simulink model "ThreeWheeledVehicle"  (R2017b)
settings: Solver=VariableStepAuto  StartTime=0.0  StopTime=25  RelTol=1e-3
undefined symbols (not defined in the file): b_contact_RW, C_F_alpha, C_F_kappa, CM_phi, Cylinder, Dtheta0, epsilon, g, k_contact_RW, lengthRW, massRW, Parts_Lib, radiusRW, sigbuilder_block, sigma, X, xPla, Y, yPla, Z, zPla
libraries: nesl_utility x42, sm_lib x39, vrlib x21, simulink x3
(part 3 of 3)

== system ThreeWheeledVehicle/Tire model1/Lateral Force A ==
  v_cx : Inport
  alpha : Inport  Port=2
  eLat : Inport  Port=3
  Constant : Constant  Value=sigma
  Constant1 : Constant  Value=sigma
  Gain : Gain  Gain=-C_F_alpha
  Integrator : Integrator
  Product{,1..4} (5 alike) : Product
  Scope : Scope
  Scope1 : Scope
  Sum : Sum  Inputs=|+-
  v_cx1 : InportShadow
  Fz : Outport
  wires:
  alpha/1 -> Scope1/1, Product/1  "input"
  v_cx/1 -> Product1/1
  Product/1 -> Sum/1
  Product1/1 -> Product/2
  Constant/1 -> Product1/2
  Sum/1 -> Integrator/1
  Integrator/1 -> Gain/1, Product2/1  "output"
  v_cx1/1 -> Product3/1
  Constant1/1 -> Product3/2
  Product3/1 -> Product2/2
  Product2/1 -> Sum/2
  Gain/1 -> Product4/1
  eLat/1 -> Product4/2
  Product4/1 -> Scope/1, Fz/1

== system ThreeWheeledVehicle/Tire model1/Lateral slip with relaxation ==
  v_s : Inport
  eLat : Inport  Port=2
  v_cx : Inport  Port=3
  eLong : Inport  Port=4
  Dot Product : DotProduct  InputSameDT=on  OutDataTypeStr=Inherit: Inherit via internal rule
  Gain : Gain  Gain=1/sigma
  Gain1 : Gain  Gain=-C_F_alpha
  Integrator : Integrator
  Product : Product
  Product1 : Product
  Scope : Scope
  Scope1 : Scope
  Scope2 : Scope
  Sum : Sum  Inputs=|+-
  F_Lat : Outport
  wires:
  v_s/1 -> Dot Product/1
  eLat/1 -> Product1/2, Dot Product/2
  Dot Product/1 -> Scope1/1, Sum/1  "s2"
  Product/1 -> Sum/2
  Sum/1 -> Gain/1
  Gain/1 -> Integrator/1
  Integrator/1 -> Scope2/1, Gain1/1, Product/2  "alpha_F"
  Gain1/1 -> Product1/1
  Product1/1 -> Scope/1, F_Lat/1
  v_cx/1 -> Product/1

== system ThreeWheeledVehicle/Tire model1/Longitudinal Force A ==
  v_cx : Inport
  kappa : Inport  Port=2
  eLong : Inport  Port=3
  Constant : Constant  Value=sigma
  Constant1 : Constant  Value=sigma
  Gain : Gain  Gain=-C_F_kappa
  Integrator : Integrator
  Product{,1..4} (5 alike) : Product
  Scope : Scope
  Scope1 : Scope
  Sum : Sum  Inputs=|+-
  v_cx1 : InportShadow
  Fx : Outport
  wires:
  kappa/1 -> Scope1/1, Product/1  "input"
  v_cx/1 -> Product1/1
  Product/1 -> Sum/1
  Product1/1 -> Product/2
  Constant/1 -> Product1/2
  Sum/1 -> Integrator/1
  Integrator/1 -> Gain/1, Product2/1  "output"
  v_cx1/1 -> Product3/1
  Constant1/1 -> Product3/2
  Product3/1 -> Product2/2
  Product2/1 -> Sum/2
  Gain/1 -> Product4/1
  eLong/1 -> Product4/2
  Product4/1 -> Scope/1, Fx/1

== system ThreeWheeledVehicle/Tire model1/Longitudinal slip with relaxation ==
  v_s : Inport
  eLong : Inport  Port=2
  v_cx : Inport  Port=3
  Dot Product : DotProduct  InputSameDT=on  OutDataTypeStr=Inherit: Inherit via internal rule
  Gain : Gain  Gain=1/sigma
  Gain1 : Gain  Gain=-C_F_kappa
  Integrator : Integrator
  Product : Product
  Product1 : Product
  Scope : Scope
  Scope1 : Scope
  Sum : Sum  Inputs=|+-
  F_Long : Outport
  wires:
  v_s/1 -> Dot Product/1
  eLong/1 -> Product1/2, Dot Product/2
  Dot Product/1 -> Scope1/1, Sum/1  "s1"
  Product/1 -> Sum/2
  Sum/1 -> Gain/1
  Gain/1 -> Integrator/1
  Integrator/1 -> Gain1/1, Product/2  "kappa_F"
  Gain1/1 -> Product1/1
  Product1/1 -> Scope/1, F_Long/1
  v_cx/1 -> Product/1

== system ThreeWheeledVehicle/Tire model1/Sensing ==
  PS-Simulink Converter{,1..9} (10 alike) : nesl_utility/PS-Simulink Converter  PhysicalDomain=network_engine_domain  SubClassName=ps_output  LeftPortType=input  RightPortType=output  PseudoPeriodic=off  Frequencies=[]  Unit=1  AffineConversion=off
  Scope : Scope
  Transform Sensor : sm_lib/Frames and Transforms/Transform Sensor  MeasurementFrame=Base  SenseAngle=off  SenseAxis=off  SenseAngle1=off  SenseAngle2=off  SenseAngle3=off  SenseQ=off  SenseR=on  SenseOmegaX=on  SenseOmegaY=on  SenseOmegaZ=on  SenseOmega1=off  SenseOmega2=off  SenseOmega3=off  SenseQDot=off  SenseRDot=off  SenseAlphaX=off  SenseAlphaY=off  SenseAlphaZ=off  SenseAlpha1=off  SenseAlpha2=off  SenseAlpha3=off  SenseQDDot=off  SenseRDDot=off  SenseX=on  SenseY=on  SenseZ=on  SenseRad=off  SenseAzim=off  SenseDist=off  SenseInc=off  SenseXDot=on  SenseYDot=on  SenseZDot=on  SenseRadDot=off  SenseAzimDot=off  SenseDistDot=off  SenseIncDot=off  SenseXDDot=off  SenseYDDot=off  SenseZDDot=off  SenseRadDDot=off  SenseAzimDDot=off  SenseDistDDot=off  SenseIncDDot=off
  Wheel : PMIOPort  Port=1  Side=Left
  Plane : PMIOPort  Port=2  Side=Left
  R : Outport
  x : Outport  Port=2
  y : Outport  Port=3
  z : Outport  Port=4
  vx : Outport  Port=5
  vy : Outport  Port=6
  vz : Outport  Port=7
  wx : Outport  Port=8
  wy : Outport  Port=9
  wz : Outport  Port=10
  wires:
  PS-Simulink Converter2/1 -> wy/1
  PS-Simulink Converter8/1 -> vy/1
  PS-Simulink Converter9/1 -> vz/1
  PS-Simulink Converter1/1 -> wx/1
  PS-Simulink Converter4/1 -> x/1
  PS-Simulink Converter7/1 -> vx/1
  PS-Simulink Converter3/1 -> wz/1
  PS-Simulink Converter5/1 -> y/1
  PS-Simulink Converter6/1 -> Scope/1, z/1
  PS-Simulink Converter/1 -> R/1
  connections:
  PS-Simulink Converter1/LConn1 -- Transform Sensor/RConn3
  PS-Simulink Converter4/LConn1 -- Transform Sensor/RConn6
  PS-Simulink Converter3/LConn1 -- Transform Sensor/RConn5
  PS-Simulink Converter9/LConn1 -- Transform Sensor/RConn11
  PS-Simulink Converter2/LConn1 -- Transform Sensor/RConn4
  PS-Simulink Converter6/LConn1 -- Transform Sensor/RConn8
  PS-Simulink Converter/LConn1 -- Transform Sensor/RConn2
  Transform Sensor/LConn1 -- Plane/RConn1
  Transform Sensor/RConn1 -- Wheel/RConn1
  PS-Simulink Converter5/LConn1 -- Transform Sensor/RConn7
  PS-Simulink Converter7/LConn1 -- Transform Sensor/RConn9
  PS-Simulink Converter8/LConn1 -- Transform Sensor/RConn10

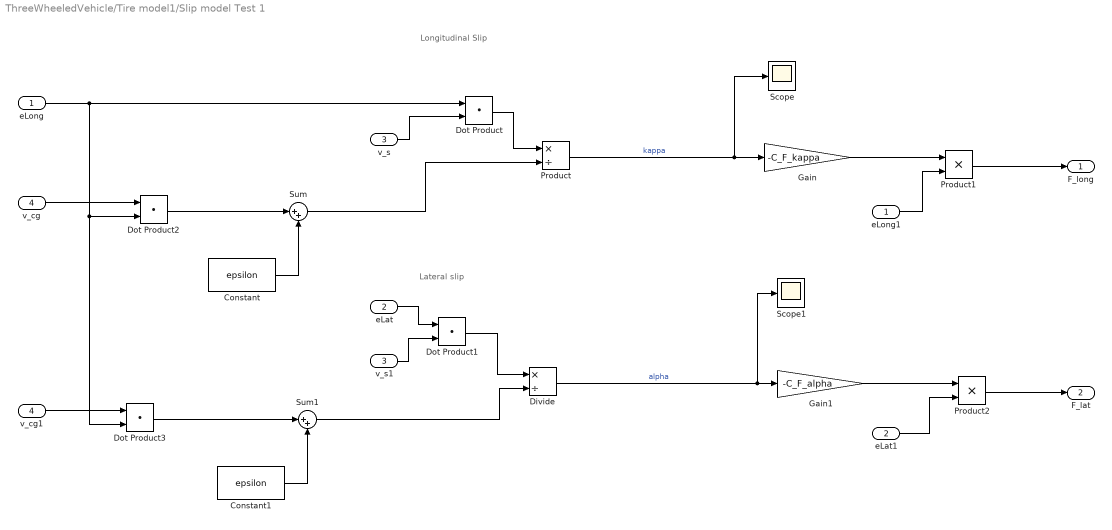
== system ThreeWheeledVehicle/Tire model1/Slip model Test 1 ==
  note: Lateral slip
  note: Longitudinal Slip
  eLong : Inport
  eLat : Inport  Port=2
  v_s : Inport  Port=3
  v_cg : Inport  Port=4
  Constant : Constant  Value=epsilon
  Constant1 : Constant  Value=epsilon
  Divide : Product  Inputs=*/
  Dot Product{,1..3} (4 alike) : DotProduct  InputSameDT=on  OutDataTypeStr=Inherit: Inherit via internal rule
  Gain : Gain  Gain=-C_F_kappa
  Gain1 : Gain  Gain=-C_F_alpha
  Product : Product  Inputs=*/
  Product1 : Product
  Product2 : Product
  Scope : Scope
  Scope1 : Scope
  Sum : Sum  Inputs=|++
  Sum1 : Sum  Inputs=|++
  eLat1 : InportShadow  Port=2
  eLong1 : InportShadow
  v_cg1 : InportShadow  Port=4
  v_s1 : InportShadow  Port=3
  F_long : Outport
  F_lat : Outport  Port=2
  wires:
  eLong/1 -> Dot Product3/2, Dot Product2/2, Dot Product/1
  v_s/1 -> Dot Product/2
  Dot Product/1 -> Product/1
  Product/1 -> Scope/1, Gain/1  "kappa"
  eLat/1 -> Dot Product1/1
  v_s1/1 -> Dot Product1/2
  Dot Product1/1 -> Divide/1
  Divide/1 -> Scope1/1, Gain1/1  "alpha"
  Gain/1 -> Product1/1
  eLong1/1 -> Product1/2
  Gain1/1 -> Product2/1
  eLat1/1 -> Product2/2
  Product1/1 -> F_long/1
  Product2/1 -> F_lat/1
  Constant/1 -> Sum/2
  Sum/1 -> Product/2
  Constant1/1 -> Sum1/2
  Sum1/1 -> Divide/2
  v_cg/1 -> Dot Product2/1
  Dot Product2/1 -> Sum/1
  v_cg1/1 -> Dot Product3/1
  Dot Product3/1 -> Sum1/1

== system ThreeWheeledVehicle/Tire model1/Slip model Test 2 ==
  note: Lateral slip
  note: Longitudinal Slip
  eLong : Inport
  eLat : Inport  Port=2
  v_s : Inport  Port=3
  v_cx : Inport  Port=4
  Divide : Product  Inputs=*/
  Dot Product : DotProduct  InputSameDT=on  OutDataTypeStr=Inherit: Inherit via internal rule
  Dot Product1 : DotProduct  InputSameDT=on  OutDataTypeStr=Inherit: Inherit via internal rule
  Gain : Gain  Gain=-C_F_kappa
  Gain1 : Gain  Gain=-C_F_alpha
  Product : Product  Inputs=*/
  Product1 : Product
  Product2 : Product
  Scope : Scope
  Scope1 : Scope
  eLat1 : InportShadow  Port=2
  eLong1 : InportShadow
  v_cx1 : InportShadow  Port=4
  v_s1 : InportShadow  Port=3
  F_long : Outport
  F_lat : Outport  Port=2
  kappa : Outport  Port=3
  alpha : Outport  Port=4
  wires:
  eLong/1 -> Dot Product/1
  Dot Product/1 -> Product/1
  eLat/1 -> Dot Product1/1
  Dot Product1/1 -> Divide/1
  Divide/1 -> alpha/1, Scope1/1, Gain1/1  "alpha"
  Gain/1 -> Product1/1
  eLong1/1 -> Product1/2
  Gain1/1 -> Product2/1
  eLat1/1 -> Product2/2
  Product1/1 -> F_long/1
  Product2/1 -> F_lat/1
  v_s/1 -> Dot Product/2
  v_s1/1 -> Dot Product1/2
  Product/1 -> Scope/1, kappa/1, Gain/1  "kappa"
  v_cx/1 -> Divide/2, Product/2

== system ThreeWheeledVehicle/Tire model1/Slip velocity ==
  omega : Inport
  v_cg : Inport  Port=2
  r : Inport  Port=3
  Add : Sum
  Cross Product : vrlib/Utilities/Cross Product
      settings: SourceProductBaseCode=VR
  Scope : Scope
  Scope1 : Scope
  Scope4 : Scope
  v_s : Outport
  wires:
  omega/1 -> Cross Product/1
  Cross Product/1 -> Scope/1, Add/2  "v_r"
  r/1 -> Cross Product/2
  Add/1 -> Scope4/1, v_s/1
  v_cg/1 -> Scope1/1, Add/1  "V_x"

== system ThreeWheeledVehicle/Tire model1/Turn Slip ==
  omega : Inport
  n : Inport  Port=2
  v_cx : Inport  Port=3
  Dot Product : DotProduct  InputSameDT=on  OutDataTypeStr=Inherit: Inherit via internal rule
  Gain : Gain  Gain=1/sigma
  Gain1 : Gain  Gain=-CM_phi
  Integrator : Integrator
  Product : Product
  Product1 : Product
  Sum : Sum  Inputs=|+-
  phi_t : Outport
  wires:
  omega/1 -> Dot Product/1
  n/1 -> Product/2, Dot Product/2
  Dot Product/1 -> Sum/1
  Sum/1 -> Gain/1
  Gain/1 -> Integrator/1
  Integrator/1 -> Product1/2, Gain1/1
  Gain1/1 -> Product/1
  Product/1 -> phi_t/1
  v_cx/1 -> Product1/1
  Product1/1 -> Sum/2

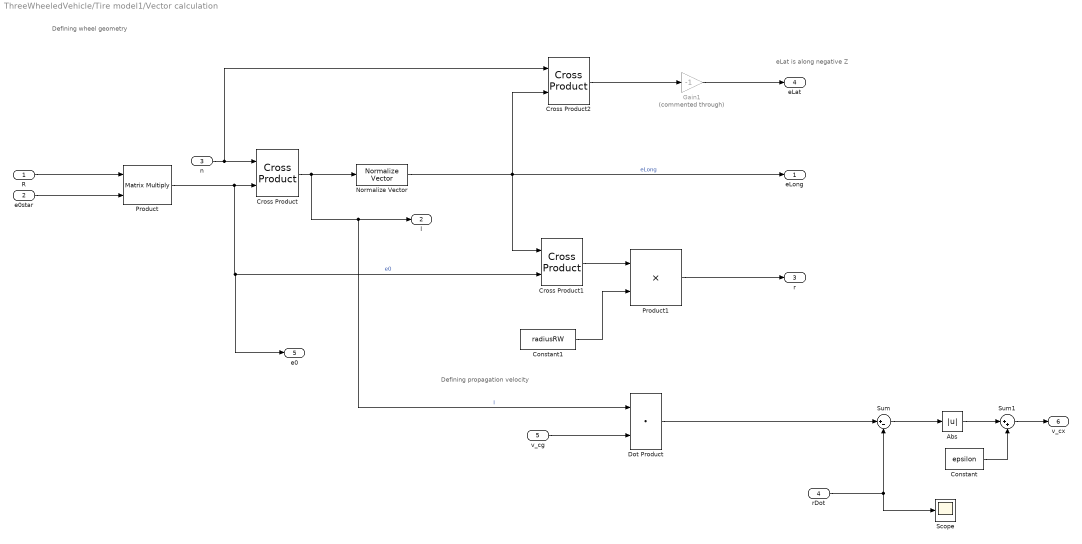
== system ThreeWheeledVehicle/Tire model1/Vector calculation ==
  note: Defining propagation velocity
  note: Defining wheel geometry
  note: eLat is along
      | negative Z
  R : Inport
  e0star : Inport  Port=2
  n : Inport  Port=3
  rDot : Inport  Port=4
  v_cg : Inport  Port=5
  Abs : Abs  ZeroCross=off
  Constant : Constant  Value=epsilon
  Constant1 : Constant  Value=radiusRW
  Cross Product : vrlib/Utilities/Cross Product
      settings: SourceProductBaseCode=VR
  Cross Product1 : vrlib/Utilities/Cross Product
      settings: SourceProductBaseCode=VR
  Cross Product2 : vrlib/Utilities/Cross Product
      settings: SourceProductBaseCode=VR
  Dot Product : DotProduct  InputSameDT=on  OutDataTypeStr=Inherit: Inherit via internal rule
  Gain1 : Gain  Commented=through  Gain=-1
  Normalize Vector : vrlib/Utilities/Normalize Vector  maxzero=0
      settings: SourceProductName=Simulink 3D Animation  SourceProductBaseCode=VR
  Product : Product  Multiplication=Matrix(*)
  Product1 : Product
  Scope : Scope
  Sum : Sum  Inputs=|+-
  Sum1 : Sum  Inputs=|++
  eLong : Outport
  l : Outport  Port=2
  r : Outport  Port=3
  eLat : Outport  Port=4
  e0 : Outport  Port=5
  v_cx : Outport  Port=6
  wires:
  R/1 -> Product/1
  e0star/1 -> Product/2
  Product/1 -> Cross Product1/2, e0/1, Cross Product/2  "e0"
  n/1 -> Cross Product2/1, Cross Product/1
  Cross Product/1 -> Dot Product/1, l/1, Normalize Vector/1  "l"
  Normalize Vector/1 -> eLong/1, Cross Product2/2, Cross Product1/1  "eLong"
  Cross Product1/1 -> Product1/1
  Cross Product2/1 -> Gain1/1
  v_cg/1 -> Dot Product/2
  Dot Product/1 -> Sum/1
  Sum/1 -> Abs/1
  Abs/1 -> Sum1/1
  Sum1/1 -> v_cx/1
  Constant/1 -> Sum1/2
  Product1/1 -> r/1
  Gain1/1 -> eLat/1
  Constant1/1 -> Product1/2
  rDot/1 -> Sum/2, Scope/1

== system ThreeWheeledVehicle/Tire model1/Verticle force ==
  note: Linear force law
  x_cg : Inport
  v_cg : Inport  Port=2
  r : Inport  Port=3
  n : Inport  Port=4
  Dot Product : DotProduct  InputSameDT=on  OutDataTypeStr=Inherit: Inherit via internal rule
  Dot Product1 : DotProduct  InputSameDT=on  OutDataTypeStr=Inherit: Inherit via internal rule
  Gain : Gain  Gain=-k_contact_RW
  Gain1 : Gain  Gain=-b_contact_RW
  Gain2 : Gain  Commented=through  Gain=-1
  Initial position of CP from ground : Constant  Value=[0 0 0]'
  Product : Product
  Scope : Scope
  Sum : Sum  Inputs=|++
  Sum1 : Sum  Inputs=|+-
  Sum2 : Sum
  Fn : Outport
  FnDisk : Outport  Port=2
  wires:
  x_cg/1 -> Sum/1
  Sum/1 -> Scope/1, Sum1/1  "CP position from ground"
  Initial position of CP from ground/1 -> Sum1/2
  Sum1/1 -> Dot Product/1
  Dot Product/1 -> Gain/1  "pen"
  v_cg/1 -> Dot Product1/2
  Dot Product1/1 -> Gain1/1  "pentration velocity"
  Gain1/1 -> Sum2/2
  Sum2/1 -> Fn/1, Gain2/1
  n/1 -> Product/2, Dot Product1/1, Dot Product/2
  Gain/1 -> Sum2/1
  r/1 -> Sum/2
  Product/1 -> FnDisk/1
  Gain2/1 -> Product/1

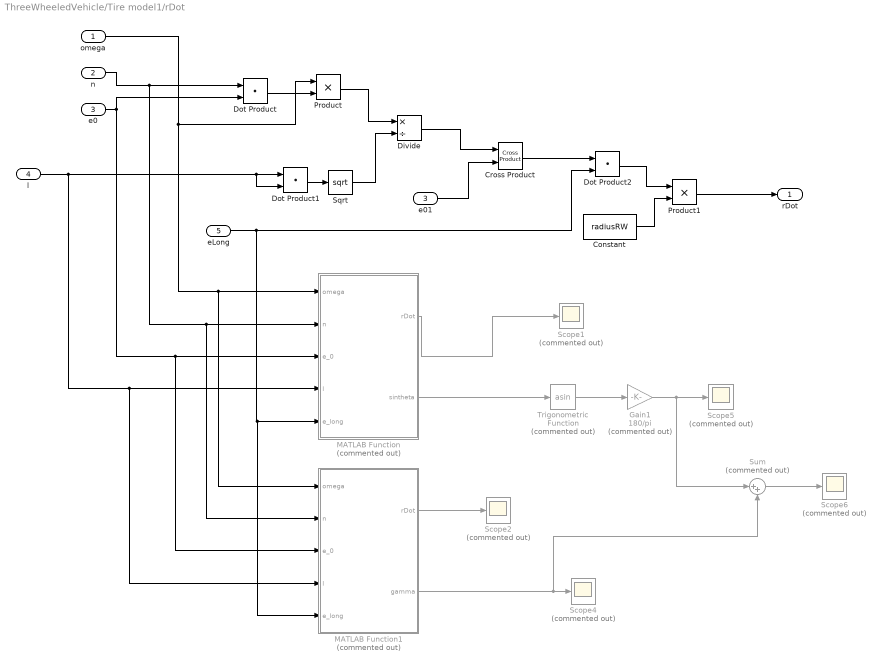
== system ThreeWheeledVehicle/Tire model1/rDot ==
  omega : Inport
  n : Inport  Port=2
  e0 : Inport  Port=3
  l : Inport  Port=4
  eLong : Inport  Port=5
  Constant : Constant  Value=radiusRW
  Cross Product : vrlib/Utilities/Cross Product
      settings: SourceProductBaseCode=VR
  Divide : Product  Inputs=*/
  Dot Product : DotProduct  InputSameDT=on  OutDataTypeStr=Inherit: Inherit via internal rule
  Dot Product1 : DotProduct  InputSameDT=on  OutDataTypeStr=Inherit: Inherit via internal rule
  Dot Product2 : DotProduct  InputSameDT=on  OutDataTypeStr=Inherit: Inherit via internal rule
  Gain1 : Gain  Commented=on  Gain=180/pi
  MATLAB Function : MATLAB Function  Commented=on  TreatAsAtomicUnit=on
  MATLAB Function1 : MATLAB Function  Commented=on  TreatAsAtomicUnit=on
  Product : Product
  Product1 : Product
  Scope{1..2,4..6} (5 alike) : Scope  Commented=on
  Sqrt : Sqrt  SaturateOnIntegerOverflow=on
  Sum : Sum  Commented=on  Inputs=|++
  Trigonometric Function : Trigonometry  Commented=on  Operator=asin
  e01 : InportShadow  Port=3
  rDot : Outport
  wires:
  n/1 -> MATLAB Function1/2(n), MATLAB Function/2(n), Dot Product/1
  e0/1 -> MATLAB Function1/3(e_0), MATLAB Function/3(e_0), Dot Product/2
  Dot Product/1 -> Product/2
  omega/1 -> MATLAB Function1/1(omega), MATLAB Function/1(omega), Product/1
  Product/1 -> Divide/1
  l/1 -> MATLAB Function1/4(l), MATLAB Function/4(l), Dot Product1/2, Dot Product1/1
  Dot Product1/1 -> Sqrt/1
  Sqrt/1 -> Divide/2
  Divide/1 -> Cross Product/1
  e01/1 -> Cross Product/2
  Cross Product/1 -> Dot Product2/1
  eLong/1 -> MATLAB Function1/5(e_long), MATLAB Function/5(e_long), Dot Product2/2
  Dot Product2/1 -> Product1/1
  Constant/1 -> Product1/2
  MATLAB Function/1(rDot) -> Scope1/1
  MATLAB Function1/1(rDot) -> Scope2/1
  Product1/1 -> rDot/1
  MATLAB Function1/2(gamma) -> Sum/2, Scope4/1
  MATLAB Function/2(sintheta) -> Trigonometric Function/1
  Trigonometric Function/1 -> Gain1/1
  Gain1/1 -> Sum/1, Scope5/1
  Sum/1 -> Scope6/1

== system ThreeWheeledVehicle/Tire model2/Camber thrust ==
  Fn : Inport
  eLat : Inport  Port=2
  n : Inport  Port=3
  e0 : Inport  Port=4
  Compare To Constant : simulink/Logic and Bit Operations/Compare To Constant  relop=<=  const=-1  OutDataTypeStr=boolean
  Dot Product : DotProduct  InputSameDT=on  OutDataTypeStr=Inherit: Inherit via internal rule
  Product : Product
  Product1 : Product
  Scope{,1..3} (4 alike) : Scope
  Stop Simulation : Stop
  camber : Outport
  wires:
  Compare To Constant/1 -> Stop Simulation/1
  Dot Product/1 -> Compare To Constant/1, Product/2, Scope2/1, Scope/1  "sin_gamma"
  Product1/1 -> camber/1, Scope1/1
  eLat/1 -> Product1/2
  e0/1 -> Dot Product/2
  n/1 -> Dot Product/1
  Product/1 -> Product1/1, Scope3/1
  Fn/1 -> Product/1

== system ThreeWheeledVehicle/Tire model2/Force and moments block ==
  F_long : Inport
  F_lat : Inport  Port=2
  FnDisk : Inport  Port=3
  r : Inport  Port=4
  R : Inport  Port=5
  camber : Inport  Port=6
  phi_t : Inport  Port=7
  Add : Sum  Inputs=4
  Add1 : Sum
  Cross Product : vrlib/Utilities/Cross Product
      settings: SourceProductBaseCode=VR
  Demux : Demux  Outputs=3
  Demux1 : Demux  Outputs=3
  Product : Product  Inputs=/*  Multiplication=Matrix(*)
  Product1 : Product  Inputs=/*  Multiplication=Matrix(*)
  Scope : Scope  NumInputPorts=3
  Scope1 : Scope  NumInputPorts=3
  F : Outport
  M : Outport  Port=2
  wires:
  phi_t/1 -> Add1/2
  r/1 -> Cross Product/1
  Product1/1 -> Demux/1, M/1
  Add1/1 -> Product1/2
  F_lat/1 -> Add/3
  F_long/1 -> Add/2
  FnDisk/1 -> Add/1
  Demux1/1 -> Scope1/1  "Fx"
  Demux1/2 -> Scope1/2  "Fy"
  Demux1/3 -> Scope1/3  "Fz"
  Product/1 -> F/1, Demux1/1
  camber/1 -> Add/4
  Cross Product/1 -> Add1/1
  Demux/1 -> Scope/1  "Mx"
  Demux/2 -> Scope/2  "My"
  Demux/3 -> Scope/3  "Mz"
  R/1 -> Product/1, Product1/1
  Add/1 -> Product/2, Cross Product/2

== system ThreeWheeledVehicle/Tire model2/Lateral Force A ==
  v_cx : Inport
  alpha : Inport  Port=2
  eLat : Inport  Port=3
  Constant : Constant  Value=sigma
  Constant1 : Constant  Value=sigma
  Gain : Gain  Gain=-C_F_alpha
  Integrator : Integrator
  Product{,1..4} (5 alike) : Product
  Scope : Scope
  Scope1 : Scope
  Sum : Sum  Inputs=|+-
  v_cx1 : InportShadow
  Fz : Outport
  wires:
  Product4/1 -> Fz/1, Scope/1
  eLat/1 -> Product4/2
  Gain/1 -> Product4/1
  Product2/1 -> Sum/2
  Product3/1 -> Product2/2
  Constant1/1 -> Product3/2
  v_cx1/1 -> Product3/1
  Integrator/1 -> Product2/1, Gain/1  "output"
  Sum/1 -> Integrator/1
  Constant/1 -> Product1/2
  Product1/1 -> Product/2
  Product/1 -> Sum/1
  v_cx/1 -> Product1/1
  alpha/1 -> Product/1, Scope1/1  "input"

== system ThreeWheeledVehicle/Tire model2/Lateral slip with relaxation ==
  v_s : Inport
  eLat : Inport  Port=2
  v_cx : Inport  Port=3
  eLong : Inport  Port=4
  Dot Product : DotProduct  InputSameDT=on  OutDataTypeStr=Inherit: Inherit via internal rule
  Gain : Gain  Gain=1/sigma
  Gain1 : Gain  Gain=-C_F_alpha
  Integrator : Integrator
  Product : Product
  Product1 : Product
  Scope : Scope
  Scope1 : Scope
  Scope2 : Scope
  Sum : Sum  Inputs=|+-
  F_Lat : Outport
  wires:
  v_cx/1 -> Product/1
  Product1/1 -> F_Lat/1, Scope/1
  Gain1/1 -> Product1/1
  Integrator/1 -> Product/2, Gain1/1, Scope2/1  "alpha_F"
  Gain/1 -> Integrator/1
  Sum/1 -> Gain/1
  Product/1 -> Sum/2
  Dot Product/1 -> Sum/1, Scope1/1  "s2"
  eLat/1 -> Dot Product/2, Product1/2
  v_s/1 -> Dot Product/1

== system ThreeWheeledVehicle/Tire model2/Longitudinal Force A ==
  v_cx : Inport
  kappa : Inport  Port=2
  eLong : Inport  Port=3
  Constant : Constant  Value=sigma
  Constant1 : Constant  Value=sigma
  Gain : Gain  Gain=-C_F_kappa
  Integrator : Integrator
  Product{,1..4} (5 alike) : Product
  Scope : Scope
  Scope1 : Scope
  Sum : Sum  Inputs=|+-
  v_cx1 : InportShadow
  Fx : Outport
  wires:
  Product4/1 -> Fx/1, Scope/1
  eLong/1 -> Product4/2
  Gain/1 -> Product4/1
  Product2/1 -> Sum/2
  Product3/1 -> Product2/2
  Constant1/1 -> Product3/2
  v_cx1/1 -> Product3/1
  Integrator/1 -> Product2/1, Gain/1  "output"
  Sum/1 -> Integrator/1
  Constant/1 -> Product1/2
  Product1/1 -> Product/2
  Product/1 -> Sum/1
  v_cx/1 -> Product1/1
  kappa/1 -> Product/1, Scope1/1  "input"

== system ThreeWheeledVehicle/Tire model2/Longitudinal slip with relaxation ==
  v_s : Inport
  eLong : Inport  Port=2
  v_cx : Inport  Port=3
  Dot Product : DotProduct  InputSameDT=on  OutDataTypeStr=Inherit: Inherit via internal rule
  Gain : Gain  Gain=1/sigma
  Gain1 : Gain  Gain=-C_F_kappa
  Integrator : Integrator
  Product : Product
  Product1 : Product
  Scope : Scope
  Scope1 : Scope
  Sum : Sum  Inputs=|+-
  F_Long : Outport
  wires:
  v_cx/1 -> Product/1
  Product1/1 -> F_Long/1, Scope/1
  Gain1/1 -> Product1/1
  Integrator/1 -> Product/2, Gain1/1  "kappa_F"
  Gain/1 -> Integrator/1
  Sum/1 -> Gain/1
  Product/1 -> Sum/2
  Dot Product/1 -> Sum/1, Scope1/1  "s1"
  eLong/1 -> Dot Product/2, Product1/2
  v_s/1 -> Dot Product/1

== system ThreeWheeledVehicle/Tire model2/Sensing ==
  PS-Simulink Converter{,1..9} (10 alike) : nesl_utility/PS-Simulink Converter  PhysicalDomain=network_engine_domain  SubClassName=ps_output  LeftPortType=input  RightPortType=output  PseudoPeriodic=off  Frequencies=[]  Unit=1  AffineConversion=off
  Scope : Scope
  Transform Sensor : sm_lib/Frames and Transforms/Transform Sensor  MeasurementFrame=Base  SenseAngle=off  SenseAxis=off  SenseAngle1=off  SenseAngle2=off  SenseAngle3=off  SenseQ=off  SenseR=on  SenseOmegaX=on  SenseOmegaY=on  SenseOmegaZ=on  SenseOmega1=off  SenseOmega2=off  SenseOmega3=off  SenseQDot=off  SenseRDot=off  SenseAlphaX=off  SenseAlphaY=off  SenseAlphaZ=off  SenseAlpha1=off  SenseAlpha2=off  SenseAlpha3=off  SenseQDDot=off  SenseRDDot=off  SenseX=on  SenseY=on  SenseZ=on  SenseRad=off  SenseAzim=off  SenseDist=off  SenseInc=off  SenseXDot=on  SenseYDot=on  SenseZDot=on  SenseRadDot=off  SenseAzimDot=off  SenseDistDot=off  SenseIncDot=off  SenseXDDot=off  SenseYDDot=off  SenseZDDot=off  SenseRadDDot=off  SenseAzimDDot=off  SenseDistDDot=off  SenseIncDDot=off
  Wheel : PMIOPort  Port=1  Side=Left
  Plane : PMIOPort  Port=2  Side=Left
  R : Outport
  x : Outport  Port=2
  y : Outport  Port=3
  z : Outport  Port=4
  vx : Outport  Port=5
  vy : Outport  Port=6
  vz : Outport  Port=7
  wx : Outport  Port=8
  wy : Outport  Port=9
  wz : Outport  Port=10
  wires:
  PS-Simulink Converter/1 -> R/1
  PS-Simulink Converter6/1 -> z/1, Scope/1
  PS-Simulink Converter5/1 -> y/1
  PS-Simulink Converter3/1 -> wz/1
  PS-Simulink Converter7/1 -> vx/1
  PS-Simulink Converter4/1 -> x/1
  PS-Simulink Converter1/1 -> wx/1
  PS-Simulink Converter9/1 -> vz/1
  PS-Simulink Converter8/1 -> vy/1
  PS-Simulink Converter2/1 -> wy/1
  connections:
  PS-Simulink Converter8/LConn1 -- Transform Sensor/RConn10
  PS-Simulink Converter7/LConn1 -- Transform Sensor/RConn9
  PS-Simulink Converter5/LConn1 -- Transform Sensor/RConn7
  Transform Sensor/RConn1 -- Wheel/RConn1
  Transform Sensor/LConn1 -- Plane/RConn1
  PS-Simulink Converter/LConn1 -- Transform Sensor/RConn2
  PS-Simulink Converter6/LConn1 -- Transform Sensor/RConn8
  PS-Simulink Converter2/LConn1 -- Transform Sensor/RConn4
  PS-Simulink Converter9/LConn1 -- Transform Sensor/RConn11
  PS-Simulink Converter3/LConn1 -- Transform Sensor/RConn5
  PS-Simulink Converter4/LConn1 -- Transform Sensor/RConn6
  PS-Simulink Converter1/LConn1 -- Transform Sensor/RConn3

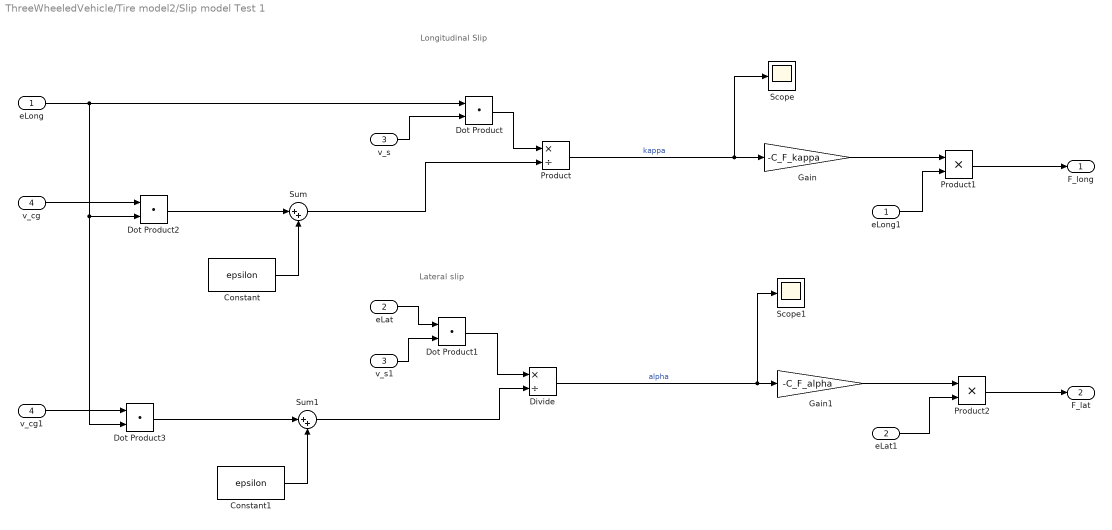
== system ThreeWheeledVehicle/Tire model2/Slip model Test 1 ==
  note: Longitudinal Slip
  note: Lateral slip
  eLong : Inport
  eLat : Inport  Port=2
  v_s : Inport  Port=3
  v_cg : Inport  Port=4
  Constant : Constant  Value=epsilon
  Constant1 : Constant  Value=epsilon
  Divide : Product  Inputs=*/
  Dot Product{,1..3} (4 alike) : DotProduct  InputSameDT=on  OutDataTypeStr=Inherit: Inherit via internal rule
  Gain : Gain  Gain=-C_F_kappa
  Gain1 : Gain  Gain=-C_F_alpha
  Product : Product  Inputs=*/
  Product1 : Product
  Product2 : Product
  Scope : Scope
  Scope1 : Scope
  Sum : Sum  Inputs=|++
  Sum1 : Sum  Inputs=|++
  eLat1 : InportShadow  Port=2
  eLong1 : InportShadow
  v_cg1 : InportShadow  Port=4
  v_s1 : InportShadow  Port=3
  F_long : Outport
  F_lat : Outport  Port=2
  wires:
  Dot Product3/1 -> Sum1/1
  v_cg1/1 -> Dot Product3/1
  Dot Product2/1 -> Sum/1
  v_cg/1 -> Dot Product2/1
  Sum1/1 -> Divide/2
  Constant1/1 -> Sum1/2
  Sum/1 -> Product/2
  Constant/1 -> Sum/2
  Product2/1 -> F_lat/1
  Product1/1 -> F_long/1
  eLat1/1 -> Product2/2
  Gain1/1 -> Product2/1
  eLong1/1 -> Product1/2
  Gain/1 -> Product1/1
  Divide/1 -> Gain1/1, Scope1/1  "alpha"
  Dot Product1/1 -> Divide/1
  v_s1/1 -> Dot Product1/2
  eLat/1 -> Dot Product1/1
  Product/1 -> Gain/1, Scope/1  "kappa"
  Dot Product/1 -> Product/1
  v_s/1 -> Dot Product/2
  eLong/1 -> Dot Product/1, Dot Product2/2, Dot Product3/2

== system ThreeWheeledVehicle/Tire model2/Slip model Test 2 ==
  note: Longitudinal Slip
  note: Lateral slip
  eLong : Inport
  eLat : Inport  Port=2
  v_s : Inport  Port=3
  v_cx : Inport  Port=4
  Divide : Product  Inputs=*/
  Dot Product : DotProduct  InputSameDT=on  OutDataTypeStr=Inherit: Inherit via internal rule
  Dot Product1 : DotProduct  InputSameDT=on  OutDataTypeStr=Inherit: Inherit via internal rule
  Gain : Gain  Gain=-C_F_kappa
  Gain1 : Gain  Gain=-C_F_alpha
  Product : Product  Inputs=*/
  Product1 : Product
  Product2 : Product
  Scope : Scope
  Scope1 : Scope
  eLat1 : InportShadow  Port=2
  eLong1 : InportShadow
  v_cx1 : InportShadow  Port=4
  v_s1 : InportShadow  Port=3
  F_long : Outport
  F_lat : Outport  Port=2
  kappa : Outport  Port=3
  alpha : Outport  Port=4
  wires:
  v_cx/1 -> Product/2, Divide/2
  Product/1 -> Gain/1, kappa/1, Scope/1  "kappa"
  v_s1/1 -> Dot Product1/2
  v_s/1 -> Dot Product/2
  Product2/1 -> F_lat/1
  Product1/1 -> F_long/1
  eLat1/1 -> Product2/2
  Gain1/1 -> Product2/1
  eLong1/1 -> Product1/2
  Gain/1 -> Product1/1
  Divide/1 -> Gain1/1, Scope1/1, alpha/1  "alpha"
  Dot Product1/1 -> Divide/1
  eLat/1 -> Dot Product1/1
  Dot Product/1 -> Product/1
  eLong/1 -> Dot Product/1

== system ThreeWheeledVehicle/Tire model2/Slip velocity ==
  omega : Inport
  v_cg : Inport  Port=2
  r : Inport  Port=3
  Add : Sum
  Cross Product : vrlib/Utilities/Cross Product
      settings: SourceProductBaseCode=VR
  Scope : Scope
  Scope1 : Scope
  Scope4 : Scope
  v_s : Outport
  wires:
  v_cg/1 -> Add/1, Scope1/1  "V_x"
  Add/1 -> v_s/1, Scope4/1
  r/1 -> Cross Product/2
  Cross Product/1 -> Add/2, Scope/1  "v_r"
  omega/1 -> Cross Product/1

== system ThreeWheeledVehicle/Tire model2/Turn Slip ==
  omega : Inport
  n : Inport  Port=2
  v_cx : Inport  Port=3
  Dot Product : DotProduct  InputSameDT=on  OutDataTypeStr=Inherit: Inherit via internal rule
  Gain : Gain  Gain=1/sigma
  Gain1 : Gain  Gain=-CM_phi
  Integrator : Integrator
  Product : Product
  Product1 : Product
  Sum : Sum  Inputs=|+-
  phi_t : Outport
  wires:
  Product1/1 -> Sum/2
  v_cx/1 -> Product1/1
  Product/1 -> phi_t/1
  Gain1/1 -> Product/1
  Integrator/1 -> Gain1/1, Product1/2
  Gain/1 -> Integrator/1
  Sum/1 -> Gain/1
  Dot Product/1 -> Sum/1
  n/1 -> Dot Product/2, Product/2
  omega/1 -> Dot Product/1

== system ThreeWheeledVehicle/Tire model2/Vector calculation ==
  note: eLat is along
      | negative Z
  note: Defining wheel geometry
  note: Defining propagation velocity
  R : Inport
  e0star : Inport  Port=2
  n : Inport  Port=3
  rDot : Inport  Port=4
  v_cg : Inport  Port=5
  Abs : Abs  ZeroCross=off
  Constant : Constant  Value=epsilon
  Constant1 : Constant  Value=radiusRW
  Cross Product : vrlib/Utilities/Cross Product
      settings: SourceProductBaseCode=VR
  Cross Product1 : vrlib/Utilities/Cross Product
      settings: SourceProductBaseCode=VR
  Cross Product2 : vrlib/Utilities/Cross Product
      settings: SourceProductBaseCode=VR
  Dot Product : DotProduct  InputSameDT=on  OutDataTypeStr=Inherit: Inherit via internal rule
  Gain1 : Gain  Commented=through  Gain=-1
  Normalize Vector : vrlib/Utilities/Normalize Vector  maxzero=0
      settings: SourceProductName=Simulink 3D Animation  SourceProductBaseCode=VR
  Product : Product  Multiplication=Matrix(*)
  Product1 : Product
  Scope : Scope
  Sum : Sum  Inputs=|+-
  Sum1 : Sum  Inputs=|++
  eLong : Outport
  l : Outport  Port=2
  r : Outport  Port=3
  eLat : Outport  Port=4
  e0 : Outport  Port=5
  v_cx : Outport  Port=6
  wires:
  rDot/1 -> Scope/1, Sum/2
  Constant1/1 -> Product1/2
  Gain1/1 -> eLat/1
  Product1/1 -> r/1
  Constant/1 -> Sum1/2
  Sum1/1 -> v_cx/1
  Abs/1 -> Sum1/1
  Sum/1 -> Abs/1
  Dot Product/1 -> Sum/1
  v_cg/1 -> Dot Product/2
  Cross Product2/1 -> Gain1/1
  Cross Product1/1 -> Product1/1
  Normalize Vector/1 -> Cross Product1/1, Cross Product2/2, eLong/1  "eLong"
  Cross Product/1 -> Normalize Vector/1, l/1, Dot Product/1  "l"
  n/1 -> Cross Product/1, Cross Product2/1
  Product/1 -> Cross Product/2, e0/1, Cross Product1/2  "e0"
  e0star/1 -> Product/2
  R/1 -> Product/1

== system ThreeWheeledVehicle/Tire model2/Verticle force ==
  note: Linear force law
  x_cg : Inport
  v_cg : Inport  Port=2
  r : Inport  Port=3
  n : Inport  Port=4
  Dot Product : DotProduct  InputSameDT=on  OutDataTypeStr=Inherit: Inherit via internal rule
  Dot Product1 : DotProduct  InputSameDT=on  OutDataTypeStr=Inherit: Inherit via internal rule
  Gain : Gain  Gain=-k_contact_RW
  Gain1 : Gain  Gain=-b_contact_RW
  Gain2 : Gain  Commented=through  Gain=-1
  Initial position of CP from ground : Constant  Value=[0 0 0]'
  Product : Product
  Scope : Scope
  Sum : Sum  Inputs=|++
  Sum1 : Sum  Inputs=|+-
  Sum2 : Sum
  Fn : Outport
  FnDisk : Outport  Port=2
  wires:
  Gain2/1 -> Product/1
  Product/1 -> FnDisk/1
  r/1 -> Sum/2
  Gain/1 -> Sum2/1
  n/1 -> Dot Product/2, Dot Product1/1, Product/2
  Sum2/1 -> Gain2/1, Fn/1
  Gain1/1 -> Sum2/2
  Dot Product1/1 -> Gain1/1  "pentration velocity"
  v_cg/1 -> Dot Product1/2
  Dot Product/1 -> Gain/1  "pen"
  Sum1/1 -> Dot Product/1
  Initial position of CP from ground/1 -> Sum1/2
  Sum/1 -> Sum1/1, Scope/1  "CP position from ground"
  x_cg/1 -> Sum/1

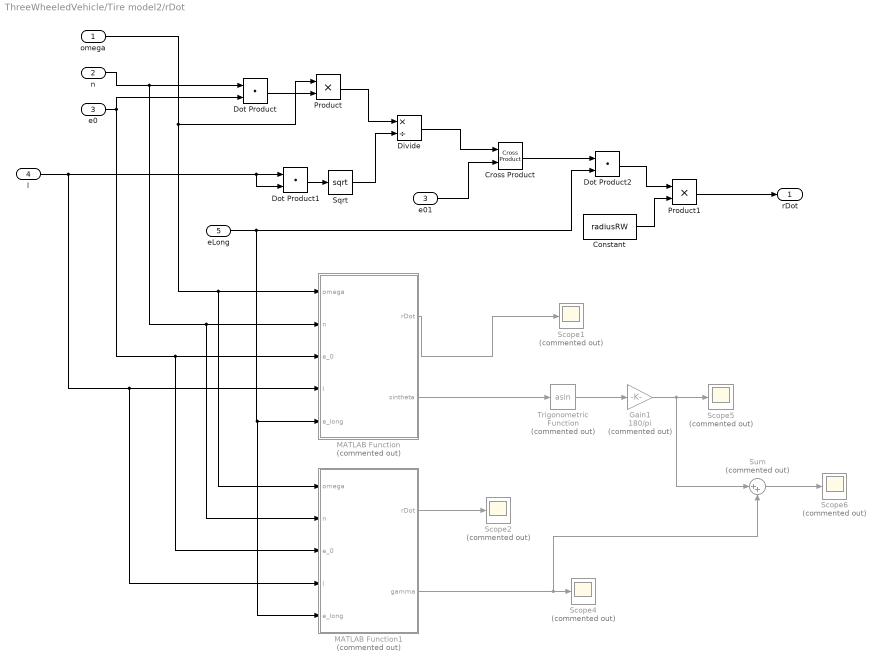
== system ThreeWheeledVehicle/Tire model2/rDot ==
  omega : Inport
  n : Inport  Port=2
  e0 : Inport  Port=3
  l : Inport  Port=4
  eLong : Inport  Port=5
  Constant : Constant  Value=radiusRW
  Cross Product : vrlib/Utilities/Cross Product
      settings: SourceProductBaseCode=VR
  Divide : Product  Inputs=*/
  Dot Product : DotProduct  InputSameDT=on  OutDataTypeStr=Inherit: Inherit via internal rule
  Dot Product1 : DotProduct  InputSameDT=on  OutDataTypeStr=Inherit: Inherit via internal rule
  Dot Product2 : DotProduct  InputSameDT=on  OutDataTypeStr=Inherit: Inherit via internal rule
  Gain1 : Gain  Commented=on  Gain=180/pi
  MATLAB Function : MATLAB Function  Commented=on  TreatAsAtomicUnit=on
  MATLAB Function1 : MATLAB Function  Commented=on  TreatAsAtomicUnit=on
  Product : Product
  Product1 : Product
  Scope{1..2,4..6} (5 alike) : Scope  Commented=on
  Sqrt : Sqrt  SaturateOnIntegerOverflow=on
  Sum : Sum  Commented=on  Inputs=|++
  Trigonometric Function : Trigonometry  Commented=on  Operator=asin
  e01 : InportShadow  Port=3
  rDot : Outport
  wires:
  Sum/1 -> Scope6/1
  Gain1/1 -> Scope5/1, Sum/1
  Trigonometric Function/1 -> Gain1/1
  MATLAB Function/2(sintheta) -> Trigonometric Function/1
  MATLAB Function1/2(gamma) -> Scope4/1, Sum/2
  Product1/1 -> rDot/1
  MATLAB Function1/1(rDot) -> Scope2/1
  MATLAB Function/1(rDot) -> Scope1/1
  Constant/1 -> Product1/2
  Dot Product2/1 -> Product1/1
  eLong/1 -> Dot Product2/2, MATLAB Function/5(e_long), MATLAB Function1/5(e_long)
  Cross Product/1 -> Dot Product2/1
  e01/1 -> Cross Product/2
  Divide/1 -> Cross Product/1
  Sqrt/1 -> Divide/2
  Dot Product1/1 -> Sqrt/1
  l/1 -> Dot Product1/1, Dot Product1/2, MATLAB Function/4(l), MATLAB Function1/4(l)
  Product/1 -> Divide/1
  omega/1 -> Product/1, MATLAB Function/1(omega), MATLAB Function1/1(omega)
  Dot Product/1 -> Product/2
  e0/1 -> Dot Product/2, MATLAB Function/3(e_0), MATLAB Function1/3(e_0)
  n/1 -> Dot Product/1, MATLAB Function/2(n), MATLAB Function1/2(n)

== matlab function ThreeWheeledVehicle/Tire model/rDot/MATLAB Function1 ==
  data: rDot output; omega input; n input; e_0 input; l input; e_long input; gamma output
function [rDot,gamma] = fcn(omega,n,e_0,l,e_long)

sinGamma = dot(n,e_0);
firstTerm = (omega*sinGamma)/norm(l);
crossProd = cross(firstTerm,e_0);
rDot = dot(crossProd,e_long);
gamma = asind(sinGamma);

== matlab function ThreeWheeledVehicle/Tire model/rDot/MATLAB Function ==
  data: rDot output; omega input; n input; e_0 input; l input; e_long input; radiusRW parameter; sintheta output
function [rDot,sintheta]  = fcn(omega,n,e_0,l,e_long, radiusRW)

sintheta = norm(l);
dotProd = dot(n,e_0);
firstTerm = omega * dotProd / sintheta;
crossProd = cross(firstTerm,e_0);
dotProd2 = dot(crossProd,e_long);
rDot = radiusRW * dotProd2;
% thetad = asind(sintheta) * (180/pi);

== matlab function ThreeWheeledVehicle/Tire model1/rDot/MATLAB Function ==
  data: rDot output; omega input; n input; e_0 input; l input; e_long input; radiusRW parameter; sintheta output
function [rDot,sintheta]  = fcn(omega,n,e_0,l,e_long, radiusRW)

sintheta = norm(l);
dotProd = dot(n,e_0);
firstTerm = omega * dotProd / sintheta;
crossProd = cross(firstTerm,e_0);
dotProd2 = dot(crossProd,e_long);
rDot = radiusRW * dotProd2;
% thetad = asind(sintheta) * (180/pi);

== matlab function ThreeWheeledVehicle/Tire model1/rDot/MATLAB Function1 ==
  data: rDot output; omega input; n input; e_0 input; l input; e_long input; gamma output
function [rDot,gamma] = fcn(omega,n,e_0,l,e_long)

sinGamma = dot(n,e_0);
firstTerm = (omega*sinGamma)/norm(l);
crossProd = cross(firstTerm,e_0);
rDot = dot(crossProd,e_long);
gamma = asind(sinGamma);

== matlab function ThreeWheeledVehicle/Tire model2/rDot/MATLAB Function ==
  data: rDot output; omega input; n input; e_0 input; l input; e_long input; radiusRW parameter; sintheta output
function [rDot,sintheta]  = fcn(omega,n,e_0,l,e_long, radiusRW)

sintheta = norm(l);
dotProd = dot(n,e_0);
firstTerm = omega * dotProd / sintheta;
crossProd = cross(firstTerm,e_0);
dotProd2 = dot(crossProd,e_long);
rDot = radiusRW * dotProd2;
% thetad = asind(sintheta) * (180/pi);

== matlab function ThreeWheeledVehicle/Tire model2/rDot/MATLAB Function1 ==
  data: rDot output; omega input; n input; e_0 input; l input; e_long input; gamma output
function [rDot,gamma] = fcn(omega,n,e_0,l,e_long)

sinGamma = dot(n,e_0);
firstTerm = (omega*sinGamma)/norm(l);
crossProd = cross(firstTerm,e_0);
rDot = dot(crossProd,e_long);
gamma = asind(sinGamma);
